simulink model "adder"  (R2021a)
settings: Solver=VariableStepAuto  StartTime=0.0  StopTime=10.0  RelTol=1e-3
libraries: simulink_extras x2
settings Model: Creator=user  LastModifiedBy=user

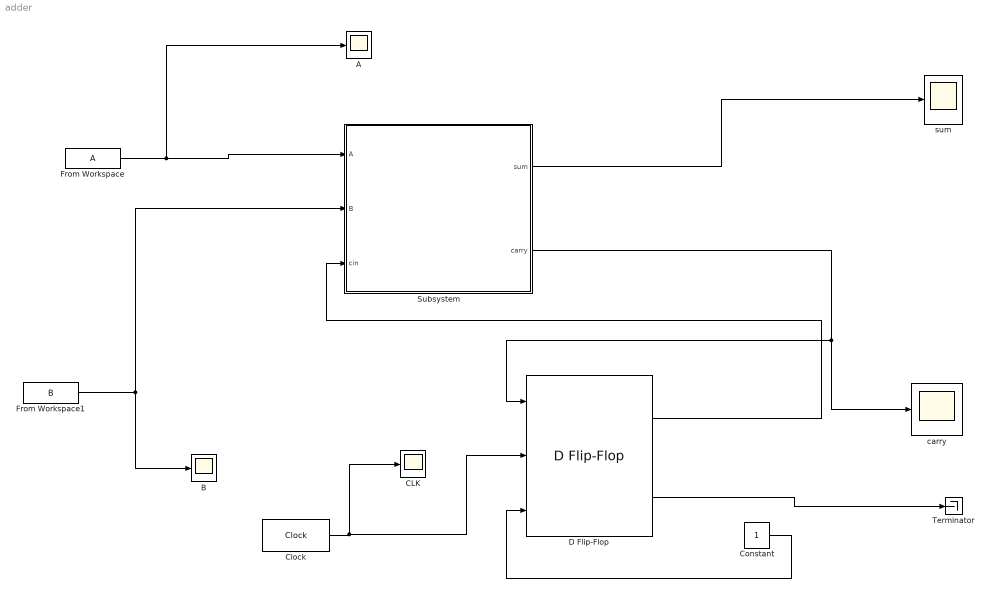
== system adder ==
  A : Scope
  B : Scope
  CLK : Scope
  Clock : simulink_extras/Flip Flops/Clock  period=1
  Constant : Constant
  D Flip-Flop : simulink_extras/Flip Flops/D Flip-Flop
  From Workspace : FromWorkspace  VariableName=A  Interpolate=off  OutputAfterFinalValue=Holding final value
  From Workspace1 : FromWorkspace  VariableName=B  Interpolate=off  OutputAfterFinalValue=Holding final value
  Subsystem : Subsystem
  Terminator : Terminator
  carry : Scope
  sum : Scope
  wires:
  From Workspace/1 -> Subsystem/1(A), A/1
  From Workspace1/1 -> Subsystem/2(B), B/1
  D Flip-Flop/2 -> Terminator/1
  Constant/1 -> D Flip-Flop/3
  Clock/1 -> D Flip-Flop/2, CLK/1
  Subsystem/2(carry) -> carry/1, D Flip-Flop/1
  D Flip-Flop/1 -> Subsystem/3(cin)
  Subsystem/1(sum) -> sum/1

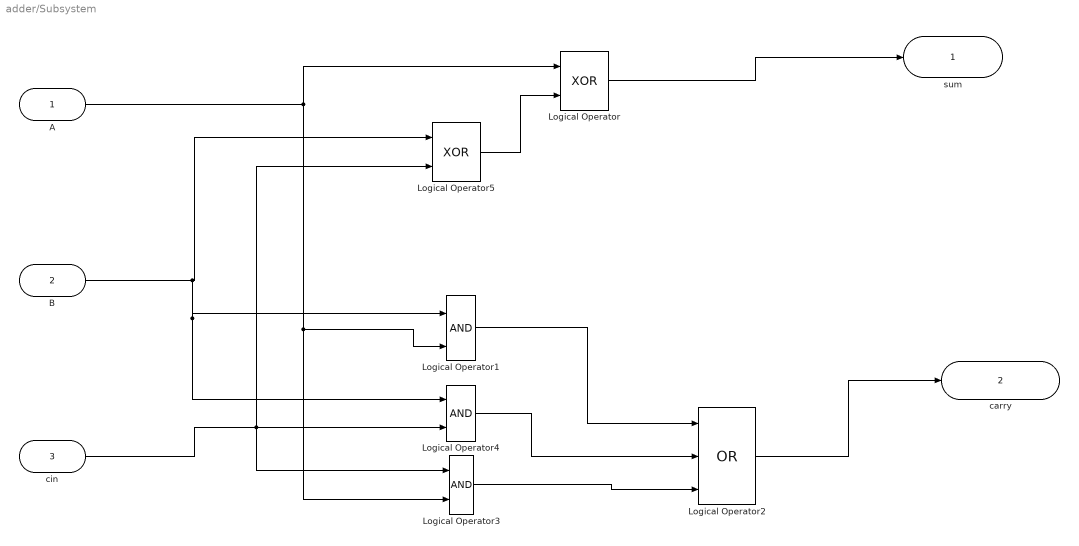
== system adder/Subsystem ==
  A : Inport
  B : Inport  Port=2
  cin : Inport  Port=3
  Logical Operator : Logic  Operator=XOR  IconShape=distinctive  AllPortsSameDT=off  OutDataTypeStr=boolean
  Logical Operator1 : Logic  IconShape=distinctive  AllPortsSameDT=off  OutDataTypeStr=boolean
  Logical Operator2 : Logic  Operator=OR  Inputs=3  IconShape=distinctive  AllPortsSameDT=off  OutDataTypeStr=boolean
  Logical Operator3 : Logic  IconShape=distinctive  AllPortsSameDT=off  OutDataTypeStr=boolean
  Logical Operator4 : Logic  IconShape=distinctive  AllPortsSameDT=off  OutDataTypeStr=boolean
  Logical Operator5 : Logic  Operator=XOR  IconShape=distinctive  AllPortsSameDT=off  OutDataTypeStr=boolean
  sum : Outport
  carry : Outport  Port=2
  wires:
  Logical Operator1/1 -> Logical Operator2/1
  Logical Operator4/1 -> Logical Operator2/2
  Logical Operator3/1 -> Logical Operator2/3
  Logical Operator5/1 -> Logical Operator/2
  A/1 -> Logical Operator/1, Logical Operator1/2, Logical Operator3/2
  B/1 -> Logical Operator4/1, Logical Operator1/1, Logical Operator5/1
  cin/1 -> Logical Operator3/1, Logical Operator5/2, Logical Operator4/2
  Logical Operator2/1 -> carry/1
  Logical Operator/1 -> sum/1
